simulink model "Test_Bench_for_the_hibrid_power_system"  (R2018a)
settings: Solver=VariableStepAuto  StartTime=0.0  StopTime=10  MaxStep=10000  RelTol=10000
undefined symbols (not defined in the file): Ion, Lithium
libraries: powerlib x3, electricdrivelib x2
settings Model: Creator=Goran Vujnovic  LastModifiedBy=Goran Vujnovic

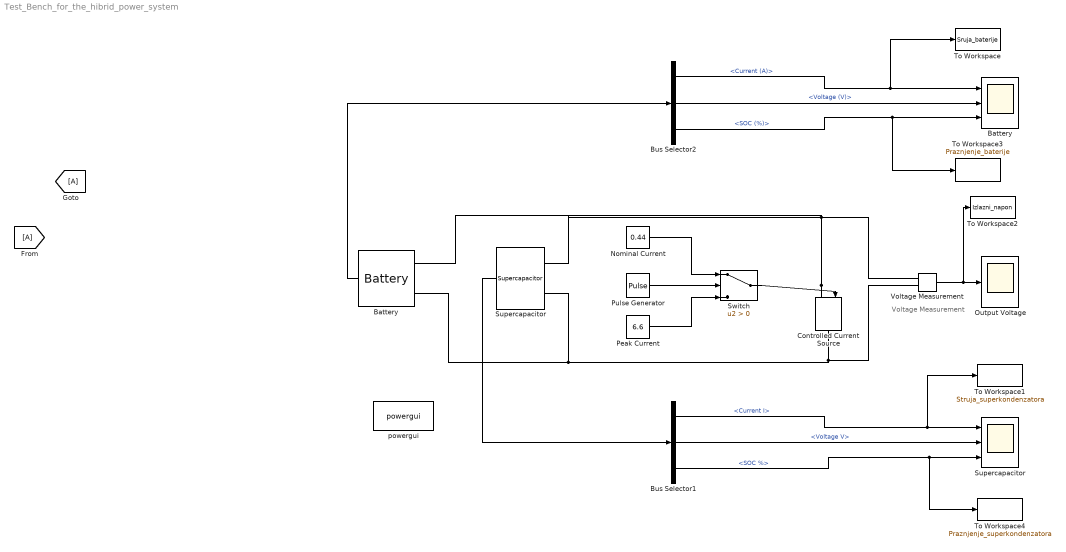
== system Test_Bench_for_the_hibrid_power_system ==
  note: Voltage Measurement
  Battery : electricdrivelib/Extra Sources/Battery  BatType=Lithium-Ion  ShowTempParam=off  ThermalPreset=no  ShowAgeParam=off  NomV=7  NomQ=5.4  SOC=100  Batt_Tr=30  PresetModel=off  MaxQ=110  MinV=24  FullV=8.3807  Dis_rate=2.3478  R=0.013333  Normal_OP=4.8835  expZone="[7.7788      0.2653]"  current=[6.5 13 32.5]  Units=Time  Tci=20  NomT=20  T2=-30  MaxQ2=4.8  FullV2=7.1  Normal_OP2=5.655  expZone2="[6.58           1]"  Rca=0.6  ti=2000  Dp=0  Neq0=0  Tsim=1e6  Ta1=25  Qeol=5.4*0.9  Reol=0.013333*1.2  Char_age=[2.3478, 3]  Dis_age=[2.3478, 10]  N1=1500  N2=10500  N3=1000  N4=1400  Ta2=45  N5=950
  "Battery " : Scope  NumInputPorts=3
  Bus Selector1 : BusSelector  OutputSignals=Current I,Voltage V,SOC %
  Bus Selector2 : BusSelector  OutputSignals=Current (A),Voltage (V),SOC (%)
  Controlled Current Source : powerlib/Electrical Sources/Controlled Current Source  Initialize=on  Source_Type=AC  Amplitude=0  Phase=0  Frequency=0  Measurements=Current
  Nominal Current : Constant  Value=0.44
  Output Voltage : Scope
  "Peak Current " : Constant  Value=6.6
  Pulse Generator : DiscretePulseGenerator  PulseType=Time based  Period=1
  Supercapacitor : electricdrivelib/Extra Sources/Supercapacitor  C=500  Rdc=8.9e-3  Voltage=48  Ns=18  Np=1  Vinit=0  Temp=25  PresetModel=off  EstParam=off  Nc=1  r=1e-9  epsilon=6.0208e-10  Ich=10  Vstern="[0.161  2.7  7.8]"  Self_dis=on  Ioc=10  Vself="[48  47.8  47.06  44.65]"  demandeplot=off  I="[10  20 100  500]"  Units=sec  Vmax=0  If=0  deltaV=0  alpha=0  sec=0
      settings: SourceProductName=Simscape Power Systems  SourceProductBaseCode=PS
  "Supercapacitor " : Scope  NumInputPorts=3
  Switch : Switch  Criteria=u2 > Threshold
  To Workspace : ToWorkspace  VariableName=Sruja_baterije  SampleTime=-1
  To Workspace1 : ToWorkspace  VariableName=Struja_superkondenzatora  SampleTime=-1
  To Workspace2 : ToWorkspace  VariableName=Izlazni_napon  SampleTime=-1
  To Workspace3 : ToWorkspace  VariableName=Praznjenje_baterije  SampleTime=-1
  To Workspace4 : ToWorkspace  VariableName=Praznjenje_superkondenzatora  SampleTime=-1
  Voltage Measurement : powerlib/Measurements/Voltage Measurement  PhasorSimulation=off  OutputType=Complex  PSBequivalent=0
  powergui : powerlib/powergui  Priority=1  SimulationMode=Discrete  SampleTime=50e-6  frequency=60  Iterations=50  frequencyindice=0  Pbase=100e6  ErrMax=1e-4  UnitsV=kV  UnitsW=MW  buscounter=0  FunctionMessages=off  echomessages=off  EnableUseOfTLC=off  CurrentSourceSwitches=off  DisableSnubberDevices=off  DisableRonSwitches=off  DisableVfSwitches=off  DisplayEquations=off  SolverType=Tustin/Backward Euler (TBE)  Interpol=off  ExternalGateDelay=off  methode=off  Ts=100  x0status=blocks  SPID=off  SwTol=0  HookPort=off  RestoreLinks=warning  ResistiveCurrentMeasurement=off  Frange=[0:2:500]  Ylog=off  Xlog=on  ShowGrid=off  save=off  variable=ZData  structure=0  ZoomFFT=off  StartTime=0.0  cycles=1  DisplayStyle=1  fundamental=60  FreqAxis=off  MaxFrequency=1000  frequencyindicesteady=1  RmsSteady=1  display=off
  wires:
  Voltage Measurement/1 -> To Workspace2/1, Output Voltage/1
  Supercapacitor/1 -> Bus Selector1/1
  Bus Selector1/2 -> "Supercapacitor "/2  "<Voltage V>"
  Battery/1 -> Bus Selector2/1
  Bus Selector2/1 -> To Workspace/1, "Battery "/1  "<Current (A)>"
  Bus Selector2/2 -> "Battery "/2  "<Voltage (V)>"
  Bus Selector2/3 -> To Workspace3/1, "Battery "/3  "<SOC (%)>"
  Bus Selector1/1 -> To Workspace1/1, "Supercapacitor "/1  "<Current I>"
  Bus Selector1/3 -> To Workspace4/1, "Supercapacitor "/3  "<SOC %>"
  Pulse Generator/1 -> Switch/2
  Nominal Current/1 -> Switch/1
  "Peak Current "/1 -> Switch/3
  Switch/1 -> Controlled Current Source/1
  connections:
  Supercapacitor/LConn2 -- Battery/LConn2 -- Voltage Measurement/LConn2 -- Controlled Current Source/RConn1
  Controlled Current Source/LConn1 -- Battery/LConn1 -- Supercapacitor/LConn1 -- Voltage Measurement/LConn1
